simulink model "fig6_58step"  (Simulink 7.1)
settings: Solver=ode45  SolverMode=SingleTasking  StartTime=0.0  StopTime=5  RelTol=1e-3  AbsTol=1e-6
libraries: simulink x2
settings Model: Creator=Office Depot  LastModifiedBy=Office Depot  ExtModeTrigMode=oneshot  ExtModeArmWhenConnect=off
settings DataIOCC: LimitDataPoints=off
settings OptimizationCC: BlockReduction=off  BooleanDataType=off
settings DebuggingCC: SaveWithParameterizedLinksMsg=none  SignalResolutionControl=TryResolveAllWithWarning  SolverPrmCheckMsg=none  MultiTaskDSMMsg=warning  MultiTaskCondExecSysMsg=none  StrictBusMsg=None
settings HardwareCC: TargetUnknown=on
settings RTWCC: IncludeERTFirstTime=on
settings STFCustomTargetCC: ModelReferenceCompliant=off  SystemTargetFile=grt.tlc

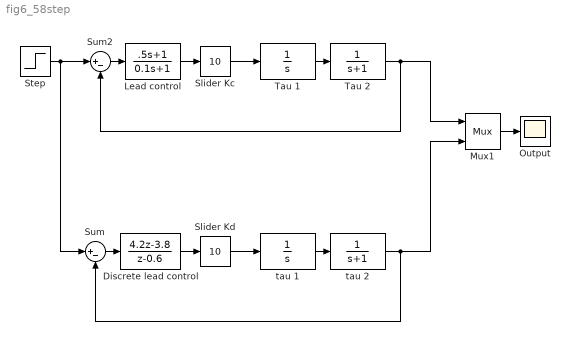
== system fig6_58step ==
  Discrete lead control : DiscreteTransferFcn  Numerator="[4.2  -3.8]"  Denominator=[1 -0.6]  SampleTime=.05
  Lead control : TransferFcn  Numerator=[.5 1]  Denominator=[0.1 1]
  Mux1 : Mux  Inputs=2
  Output : Scope
      settings: TickLabels=on  SaveName=ycd  DataFormat=Array
  Slider Kc : simulink/Math Operations/Slider Gain  SystemSampleTime=-1  low=0  gain=10  high=20
  Slider Kd : simulink/Math Operations/Slider Gain  SystemSampleTime=-1  low=0  gain=10  high=20
  Step : Step  Time=0  SampleTime=.001
  Sum : Sum  Inputs=|+-  InputSameDT=on  OutDataTypeStr=Inherit: Same as first input
  Sum2 : Sum  Inputs=|+-  InputSameDT=on  OutDataTypeStr=Inherit: Same as first input
  Tau 1 : TransferFcn  Numerator=1  Denominator=[1 0]
  Tau 2 : TransferFcn  Numerator=1  Denominator=[1 1]
  tau 1 : TransferFcn  Numerator=1  Denominator=[1 0]
  tau 2 : TransferFcn  Numerator=1  Denominator=[1 1]
  wires:
  Lead control/1 -> Slider Kc/1
  Sum2/1 -> Lead control/1
  Tau 1/1 -> Tau 2/1
  Discrete lead control/1 -> Slider Kd/1
  tau 1/1 -> tau 2/1
  Step/1 -> Sum2/1, Sum/1
  Tau 2/1 -> Mux1/1, Sum2/2
  Mux1/1 -> Output/1
  Sum/1 -> Discrete lead control/1
  tau 2/1 -> Mux1/2, Sum/2
  Slider Kc/1 -> Tau 1/1
  Slider Kd/1 -> tau 1/1
